simulink model "Stateflow_statebacktracking"  (R2015b)
settings: Solver=VariableStepAuto  StartTime=0.0  StopTime=10.0  RelTol=1e-3
settings Model: Creator=amyyang  LastModifiedBy=amyyang

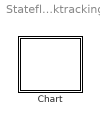
== system Stateflow_statebacktracking ==
  Chart : Stateflow chart  TreatAsAtomicUnit=on

== stateflow chart Stateflow_statebacktracking/Chart ==
  note: 不可以把复杂条件用Junction分开
  state Correct
  state InCorrect1
  state ?
  state ?
  state Correct1
  state Correct2
  note: Diagnostics诊断配置 Stateflow可以配置检查 Unexpected backtracking
  note: 不允许，否则当 CI==ON，而C2 == OFF，就会产生
      | Backtracking
  state InCorrect9
  state Correct7
  state Correct3
  state Correct4
  state Correct5
  state Correct8
  note: 所有的Junction都有分支
  state Correct6
  state Correct12
  state Correct9
  state Correct13
  state Correct10
  note: 跟左边是等效的
  state Correct14
  state Correct11
  state Correct18
  state Correct19
  state Correct16
  state InCorrect21
  state Correct15
  state Correct23
  note: 跟左边是等效的
  note: 这样就会产生回流
  state Correct20
  state Correct17
  state Correct22
  state InCorrect24
  state Correct27
  note: 比如这种形式，就要改成左边
  state Correct25
  state Correct26
  Correct -> ? : [ Condition1 && Condition2]
  InCorrect1 -> (junction 85) : [ Condition1 ]
  (junction 85) -> ? : [ Condition2 ]
  Correct1 -> Correct2 [order 2]
  Correct1 -> (junction 92) [order 1]
  (junction 92) -> (junction 93) [order 1] : [ (C1 == ON) && ( C2 == ON)]
  (junction 92) -> Correct3 [order 2] : [ Condition2]
      | {
      |  out = 1;
      | }
  (junction 93) -> Correct3 : {
      |  out = 2;
      | }
  InCorrect9 -> Correct7 [order 2] : [Condition3]
  InCorrect9 -> (junction 122) [order 1]
  (junction 122) -> (junction 123) [order 1] : [ (C1 == ON) ]
  (junction 123) -> (junction 117) : [ ( C2 == ON)]
  (junction 122) -> Correct8 [order 2] : [ Condition2]
      | {
      |  out = 1;
      | }
  (junction 117) -> Correct8 : {
      |  out = 3;
      | }
  Correct4 -> Correct5 [order 2] : [Condition3]
  Correct4 -> (junction 105) [order 1]
  (junction 105) -> (junction 108) [order 1] : [ (C1 == ON) ]
  (junction 108) -> (junction 109) [order 2] : [ ( C2 == ON)]
  (junction 105) -> Correct6 [order 2] : [ Condition2]
      | {
      |  out = 1;
      | }
  (junction 108) -> Correct6 [order 1] : {
      |  out = 2;
      | }
  (junction 109) -> Correct6 : {
      |  out = 3;
      | }
  Correct12 -> Correct13 [order 1] : [Condition3]
  Correct9 -> Correct10 [order 2] : [Condition3]
  Correct12 -> Correct14 [order 2] : [ (C1 == ON) && ( C2 == ON)]
      | {
      |  out = 2;
      | }
  Correct9 -> (junction 151) [order 1]
  (junction 151) -> (junction 154) : [ (C1 == ON) && ( C2 == ON)]
  (junction 154) -> Correct11 : {
      |  out = 2;
      | }
  Correct18 -> Correct19 [order 2] : [Condition3]
  Correct16 -> Correct15 [order 2] : [Condition3]
  InCorrect21 -> Correct23 [order 2] : [Condition3]
  Correct18 -> (junction 182) [order 1] : [ (C1 == ON) ]
  Correct16 -> (junction 167) [order 1]
  InCorrect21 -> (junction 194) [order 1]
  (junction 167) -> (junction 171) : [ (C1 == ON) ]
  (junction 194) -> (junction 205) : [ (C1 == ON) ]
  (junction 182) -> (junction 189) [order 2] : [ ( C2 == ON)]
  (junction 171) -> (junction 178) [order 2] : [ ( C2 == ON)]
  (junction 205) -> (junction 197) : [ ( C2 == ON)]
  (junction 182) -> Correct20 [order 1] : {
      |  out = 2;
      | }
  (junction 171) -> Correct17 [order 1] : {
      |  out = 2;
      | }
  (junction 189) -> Correct20 : {
      |  out = 3;
      | }
  (junction 178) -> Correct17 : {
      |  out = 3;
      | }
  (junction 197) -> Correct22 : {
      |  out = 3;
      | }
  InCorrect24 -> (junction 209) [order 1]
  InCorrect24 -> (junction 217) [order 2] : [Condition3]
  Correct27 -> (junction 226) [order 1]
  Correct27 -> (junction 227) [order 2] : [Condition3 && ( C2 == ON)]
  (junction 209) -> (junction 217) : [ (C1 == ON) ]
  (junction 217) -> (junction 214) : [ ( C2 == ON)]
  (junction 214) -> Correct25 : {
      |  out = 3;
      | }
  (junction 226) -> (junction 227) : [ (C1 == ON) && ( C2 == ON) ]
  (junction 227) -> Correct26 : {
      |  out = 3;
      | }
